simulink model "LeadVehicle_Module"  (R2026a)
settings: Solver=VariableStepAuto  StopTime=30
libraries: simulink x1
settings Model: Creator=ADMIN  LastModifiedBy=ASUS

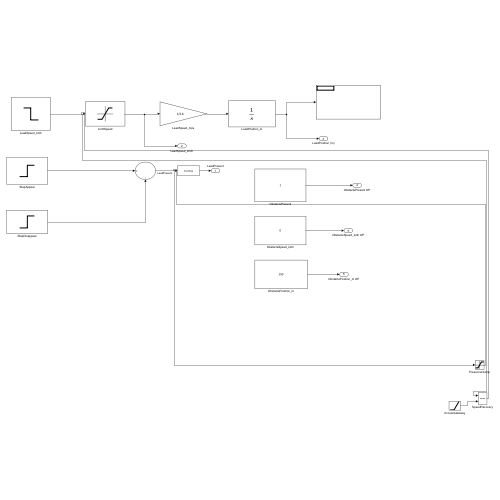
[thumbnail: Simulink's stored preview of the top-level diagram]
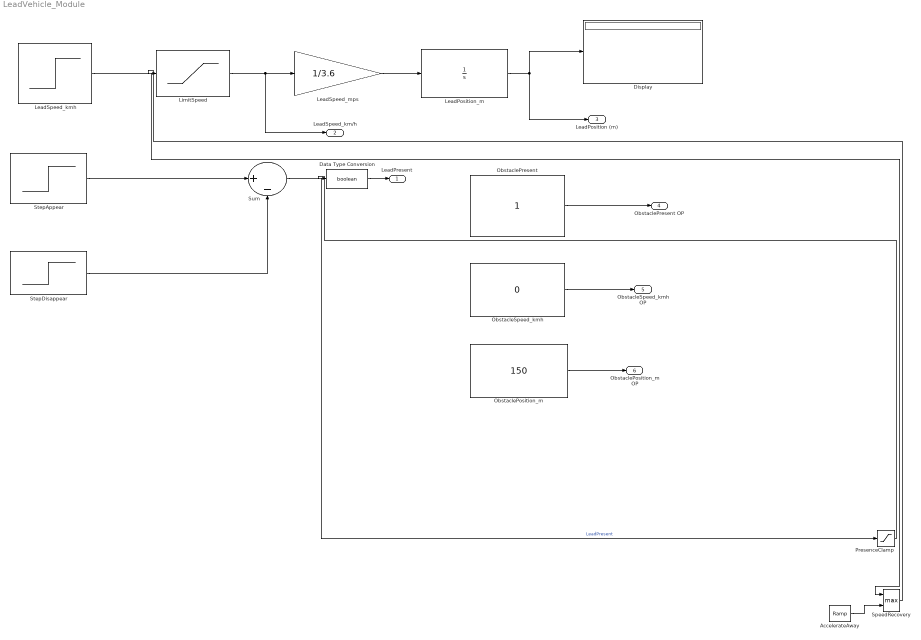
== system LeadVehicle_Module ==
  AccelerateAway : simulink/Sources/Ramp  slope=15  start=20  InitialOutput=0
  Data Type Conversion : DataTypeConversion  OutDataTypeStr=boolean  SaturateOnIntegerOverflow=off  RndMeth=Floor
  Display : Display
  LeadPosition_m : Integrator  InitialCondition=60
  LeadSpeed_kmh : Step  Time=15  InitialValue=50  FinalValue=0  SampleTime=0
  LeadSpeed_mps : Gain  Gain=1/3.6
  LimitSpeed : Saturate  UpperLimit=inf  LowerLimit=0
  ObstaclePosition_m : Constant  Value=150
  ObstaclePresent : Constant
  ObstacleSpeed_kmh : Constant  Value=0
  PresenceClamp : Saturate  UpperLimit=inf  LowerLimit=0
  SpeedRecovery : MinMax  Function=max  Inputs=2
  StepAppear : Step  Time=5  SampleTime=0
  StepDisappear : Step  Time=25  SampleTime=0
  Sum : Sum  Inputs=|+-
  LeadPresent : Outport
  LeadSpeed_km/h : Outport  Port=2
  LeadPosition (m) : Outport  Port=3
  ObstaclePresent OP : Outport  Port=4
  ObstacleSpeed_kmh OP : Outport  Port=5
  ObstaclePosition_m OP : Outport  Port=6
  wires:
  LimitSpeed/1 -> LeadSpeed_km/h/1, LeadSpeed_mps/1
  LeadSpeed_mps/1 -> LeadPosition_m/1
  StepAppear/1 -> Sum/1
  StepDisappear/1 -> Sum/2
  LeadPosition_m/1 -> LeadPosition (m)/1, Display/1
  ObstaclePresent/1 -> ObstaclePresent OP/1
  ObstacleSpeed_kmh/1 -> ObstacleSpeed_kmh OP/1
  ObstaclePosition_m/1 -> ObstaclePosition_m OP/1
  Data Type Conversion/1 -> LeadPresent/1
  Sum/1 -> PresenceClamp/1  "LeadPresent"
  PresenceClamp/1 -> Data Type Conversion/1
  LeadSpeed_kmh/1 -> SpeedRecovery/1
  AccelerateAway/1 -> SpeedRecovery/2
  SpeedRecovery/1 -> LimitSpeed/1
